simulink model "OpenFAST_ROSCO_LDP_FFP_MMPC"  (R2025b)
settings: Solver=ode4  StartTime=0.0  StopTime=TMax  FixedStep=DT  RelTol=1e-3
values from neighbouring files (symbols this model uses):
  P = P_horizon    (= 12)    [GetMPC.m]    (also in RunExample_Simulink.m = ReadWrite_FAST(fast))
undefined symbols (not defined in the file or in its folder): F, GetFASTPar, LDP, OutList, R, simu, strmatch
libraries: simulink x1
settings Model: LastModifiedBy=Aravind
settings OptimizationCC: BlockReduction=off  BooleanDataType=off
settings DebuggingCC: SaveWithParameterizedLinksMsg=none  UnderspecifiedInitializationDetection=Classic  MergeDetectMultiDrivingBlocksExec=none  SignalResolutionControl=TryResolveAllWithWarning  UnconnectedInputMsg=warning  UnconnectedOutputMsg=warning  UnconnectedLineMsg=warning
settings HardwareCC: TargetUnknown=on
settings ModelReferenceCC: EnableRefExpFcnMdlSchedulingChecks=on  PropagateSignalLabelsOutOfModel=off
settings RTWCC: GPUComputeCapability=3.5  DLArmComputeVersion=19.05

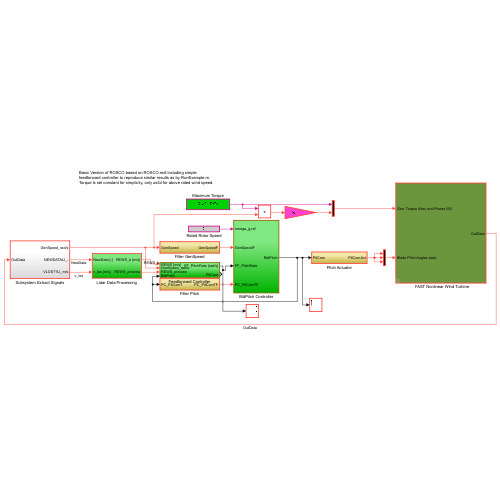
[thumbnail: Simulink's stored preview of the top-level diagram]
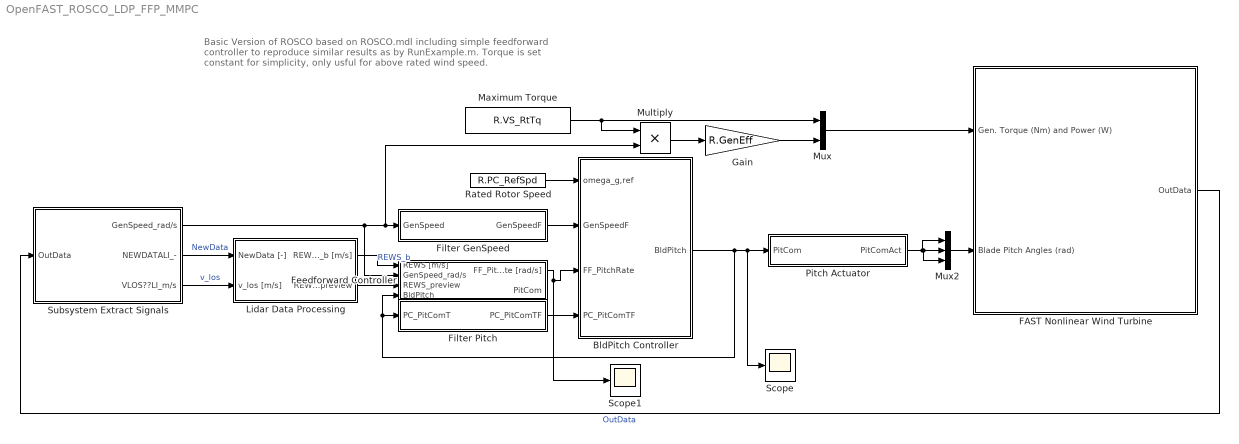
== system OpenFAST_ROSCO_LDP_FFP_MMPC ==
  note: Basic Version of ROSCO based on ROSCO.mdl including simple feedforward controller to reproduce similar results as by RunExample.m.
      | Torque is set constant for simplicity, only usful for above rated wind speed.
  "  FAST Nonlinear Wind Turbine" : Subsystem  mask(FAST Nonlinear Wind Turbine){}
      mask help: This block contains the FAST S-Function.
      mask init:
      | clear FAST_SFunc
  BldPitch Controller : Subsystem
  Feedforward Controller : Subsystem
  Filter GenSpeed : Subsystem
  Filter Pitch : Subsystem
  Gain : Gain  Gain=R.GenEff
  Lidar Data Processing : Subsystem
  Maximum Torque : Constant  Value=R.VS_RtTq
  Multiply : Product
  Mux : Mux  Inputs=2
  Mux2 : Mux  Inputs=3
  Pitch Actuator : Subsystem
  Rated Rotor Speed : Constant  Value=R.PC_RefSpd
  Scope : Scope
      settings: ActiveDisplayYMinimum=0.10219557470092069  ActiveDisplayYMaximum=0.28374092116775795  DataLoggingVariableName=ScopeData7
  Scope1 : Scope
      settings: ActiveDisplayYMinimum=-4.5750000000000979  ActiveDisplayYMaximum=4.5750000000000979  DataLoggingVariableName=ScopeData8
  Subsystem Extract Signals : Subsystem
  wires:
  Mux2/1 -> "  FAST Nonlinear Wind Turbine"/2(Blade Pitch Angles (rad))
  Rated Rotor Speed/1 -> BldPitch Controller/1(omega_g,ref)
  Subsystem Extract Signals/1(GenSpeed_rad/s) -> Feedforward Controller/2(GenSpeed_rad/s), Multiply/2, Filter GenSpeed/1(GenSpeed)
  Maximum Torque/1 -> Mux/1, Multiply/1
  Filter GenSpeed/1(GenSpeedF) -> BldPitch Controller/2(GenSpeedF)
  Gain/1 -> Mux/2
  Mux/1 -> "  FAST Nonlinear Wind Turbine"/1(Gen. Torque (Nm) and Power (W))
  Multiply/1 -> Gain/1
  "  FAST Nonlinear Wind Turbine"/1(OutData) -> Subsystem Extract Signals/1(OutData)  "OutData"
  Filter Pitch/1(PC_PitComTF) -> BldPitch Controller/4(PC_PitComTF)
  Pitch Actuator/1(PitComAct) -> Mux2/1, Mux2/3, Mux2/2
  Feedforward Controller/1(FF_PitchRate [rad/s]) -> Scope1/1, BldPitch Controller/3(FF_PitchRate)
  Subsystem Extract Signals/3(VLOS??LI_m/s) -> Lidar Data Processing/2(v_los [m/s])  "v_los"
  Lidar Data Processing/1(REWS_b [m/s]) -> Feedforward Controller/1(REWS [m/s])  "REWS_b"
  Subsystem Extract Signals/2(NEWDATALI_-) -> Lidar Data Processing/1(NewData [-])  "NewData"
  BldPitch Controller/1(BldPitch) -> Pitch Actuator/1(PitCom), Scope/1, Feedforward Controller/4(BldPitch), Filter Pitch/1(PC_PitComT)
  Lidar Data Processing/2(REWS_preview) -> Feedforward Controller/3(REWS_preview)

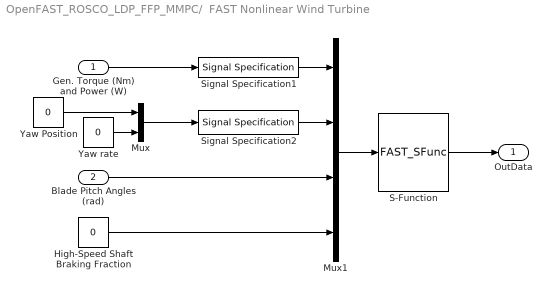
== system OpenFAST_ROSCO_LDP_FFP_MMPC/  FAST Nonlinear Wind Turbine ==
  Gen. Torque (Nm) and Power (W) : Inport
  Blade Pitch Angles (rad) : Inport  Port=2
  High-Speed Shaft Braking Fraction : Constant  Value=0
  Mux : Mux  Inputs=2
  Mux1 : Mux
  S-Function : S-Function  FunctionName=FAST_SFunc  Parameters=FAST_InputFileName, TMax, 0  SFunctionDeploymentMode=off  EnableBusSupport=off
  Signal Specification1 : SignalSpecification  OutDataTypeStr=double  Dimensions=2
  Signal Specification2 : SignalSpecification  OutDataTypeStr=double  Dimensions=2
  Yaw Position : Constant  Value=0
  Yaw rate : Constant  Value=0
  OutData : Outport
  wires:
  Gen. Torque (Nm) and Power (W)/1 -> Signal Specification1/1
  S-Function/1 -> OutData/1
  Mux1/1 -> S-Function/1
  Blade Pitch Angles (rad)/1 -> Mux1/3
  Signal Specification1/1 -> Mux1/1
  Signal Specification2/1 -> Mux1/2
  High-Speed Shaft Braking Fraction/1 -> Mux1/4
  Yaw rate/1 -> Mux/2
  Mux/1 -> Signal Specification2/1
  Yaw Position/1 -> Mux/1

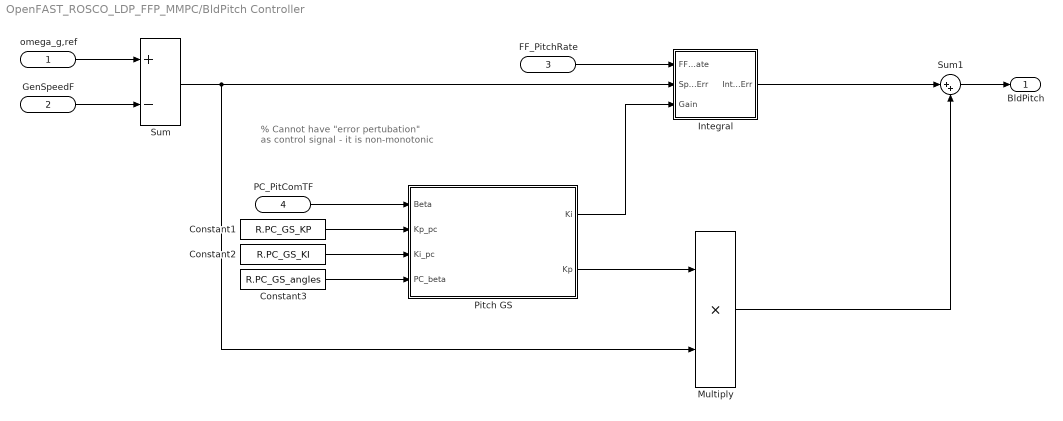
== system OpenFAST_ROSCO_LDP_FFP_MMPC/BldPitch Controller ==
  note: % Cannot have "error pertubation" as control signal
      | - it is non-monotonic
  omega_g,ref : Inport
  GenSpeedF : Inport  Port=2
  FF_PitchRate : Inport  Port=3
  PC_PitComTF : Inport  Port=4
  Constant1 : Constant  Value=R.PC_GS_KP
  Constant2 : Constant  Value=R.PC_GS_KI
  Constant3 : Constant  Value=R.PC_GS_angles
  Integral : Subsystem
  Multiply : Product
  Pitch GS : MATLAB Function  TreatAsAtomicUnit=on
  Sum : Sum  Inputs=+-
  Sum1 : Sum  Inputs=|++
  BldPitch : Outport  VectorParamsAs1DForOutWhenUnconnected=off
  wires:
  Pitch GS/1(Ki) -> Integral/3(Gain)
  omega_g,ref/1 -> Sum/1
  GenSpeedF/1 -> Sum/2
  Constant1/1 -> Pitch GS/2(Kp_pc)
  Constant2/1 -> Pitch GS/3(Ki_pc)
  Constant3/1 -> Pitch GS/4(PC_beta)
  Sum/1 -> Multiply/2, Integral/2(SpeedErr)
  Multiply/1 -> Sum1/2
  Integral/1(IntSpdErr) -> Sum1/1
  Sum1/1 -> BldPitch/1
  PC_PitComTF/1 -> Pitch GS/1(Beta)
  FF_PitchRate/1 -> Integral/1(FF_PitchRate)
  Pitch GS/2(Kp) -> Multiply/1

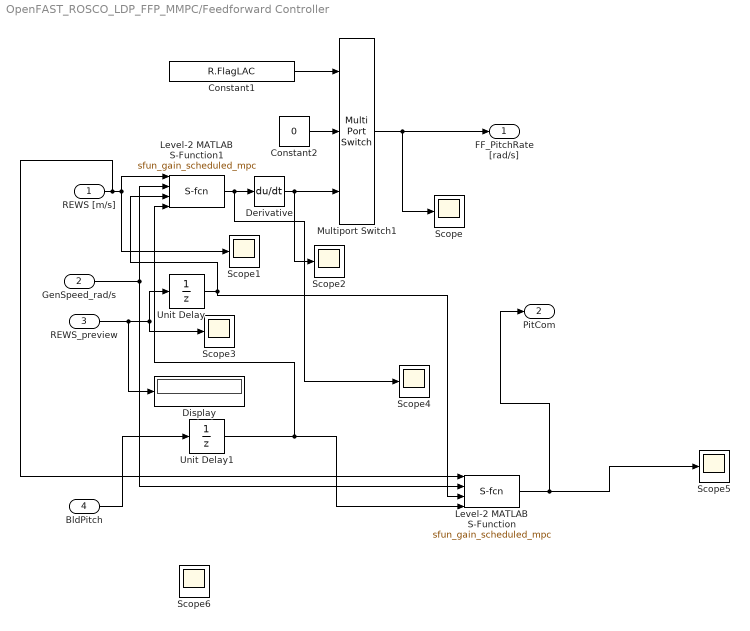
== system OpenFAST_ROSCO_LDP_FFP_MMPC/Feedforward Controller ==
  REWS [m/s] : Inport
  GenSpeed_rad/s : Inport  Port=2
  REWS_preview : Inport  Port=3
  BldPitch : Inport  Port=4
  Constant1 : Constant  Value=R.FlagLAC
  Constant2 : Constant  Value=0
  Derivative : Derivative
  Display : Display
  Level-2 MATLAB S-Function : M-S-Function  FunctionName=sfun_gain_scheduled_mpc
  Level-2 MATLAB S-Function1 : M-S-Function  FunctionName=sfun_gain_scheduled_mpc
  Multiport Switch1 : MultiPortSwitch  DataPortOrder=Specify indices  Inputs=2  DataPortIndices={0,1}  SaturateOnIntegerOverflow=off  InputSameDT=off
  Scope{,1..6} (7 alike) : Scope
      Scope settings: ActiveDisplayYMinimum=-1  ActiveDisplayYMaximum=1
      Scope1 settings: ActiveDisplayYMinimum=11.456487567346162  ActiveDisplayYMaximum=18.381466486088822  DataLoggingVariableName=ScopeData3
      Scope2 settings: ActiveDisplayYMinimum=-4.318116348637111  ActiveDisplayYMaximum=24.176537439845262  DataLoggingVariableName=ScopeData4
      Scope3 settings: ActiveDisplayYMinimum=6.7699074233965248  ActiveDisplayYMaximum=17.93615464129396  DataLoggingVariableName=ScopeData5
      Scope4 settings: ActiveDisplayYMinimum=0.080794857234064738  ActiveDisplayYMaximum=0.28427885429489819  DataLoggingVariableName=ScopeData6
      Scope5 settings: DataLoggingVariableName=ScopeData9
      Scope6 settings: DataLoggingVariableName=ScopeData10
  Unit Delay : UnitDelay  SampleTime=-1  HasFrameUpgradeWarning=on
  Unit Delay1 : UnitDelay  InitialCondition=0.1276  SampleTime=0.01  HasFrameUpgradeWarning=on
  FF_PitchRate [rad/s] : Outport  VectorParamsAs1DForOutWhenUnconnected=off
  PitCom : Outport  Port=2
  wires:
  Multiport Switch1/1 -> Scope/1, FF_PitchRate [rad/s]/1
  Constant1/1 -> Multiport Switch1/1
  Constant2/1 -> Multiport Switch1/2
  REWS [m/s]/1 -> Level-2 MATLAB S-Function/1, Level-2 MATLAB S-Function1/1, Scope1/1
  Derivative/1 -> Scope2/1, Multiport Switch1/3
  Level-2 MATLAB S-Function1/1 -> Scope4/1, Derivative/1
  GenSpeed_rad/s/1 -> Level-2 MATLAB S-Function/2, Level-2 MATLAB S-Function1/2
  REWS_preview/1 -> Scope3/1, Unit Delay/1, Display/1
  Unit Delay/1 -> Level-2 MATLAB S-Function1/3, Level-2 MATLAB S-Function/3
  BldPitch/1 -> Unit Delay1/1
  Level-2 MATLAB S-Function/1 -> PitCom/1, Scope5/1
  Unit Delay1/1 -> Level-2 MATLAB S-Function1/4, Level-2 MATLAB S-Function/4

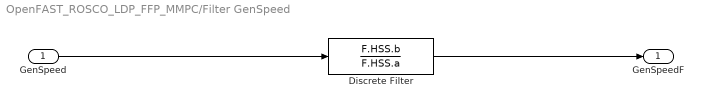
== system OpenFAST_ROSCO_LDP_FFP_MMPC/Filter GenSpeed ==
  GenSpeed : Inport
  Discrete Filter : DiscreteFilter  Numerator=F.HSS.b  Denominator=F.HSS.a  InitialStates=R.PC_RefSpd/(sum(F.HSS.a(2:end))+1)
  GenSpeedF : Outport  VectorParamsAs1DForOutWhenUnconnected=off
  wires:
  Discrete Filter/1 -> GenSpeedF/1
  GenSpeed/1 -> Discrete Filter/1

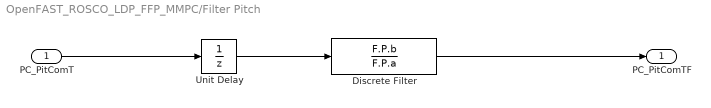
== system OpenFAST_ROSCO_LDP_FFP_MMPC/Filter Pitch ==
  PC_PitComT : Inport
  Discrete Filter : DiscreteFilter  Numerator=F.P.b  Denominator=F.P.a
  Unit Delay : UnitDelay  SampleTime=-1  HasFrameUpgradeWarning=on
  PC_PitComTF : Outport  VectorParamsAs1DForOutWhenUnconnected=off
  wires:
  PC_PitComT/1 -> Unit Delay/1
  Discrete Filter/1 -> PC_PitComTF/1
  Unit Delay/1 -> Discrete Filter/1

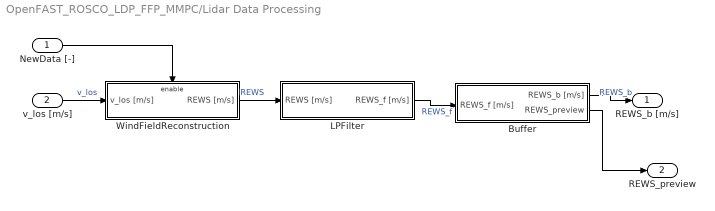
== system OpenFAST_ROSCO_LDP_FFP_MMPC/Lidar Data Processing ==
  NewData [-] : Inport
  v_los [m/s] : Inport  Port=2
  Buffer : Subsystem
  LPFilter : Subsystem
  WindFieldReconstruction : Subsystem
  REWS_b [m/s] : Outport  VectorParamsAs1DForOutWhenUnconnected=off
  REWS_preview : Outport  Port=2
  wires:
  v_los [m/s]/1 -> WindFieldReconstruction/1(v_los [m/s])  "v_los"
  NewData [-]/1 -> WindFieldReconstruction/Enable
  Buffer/1(REWS_b [m/s]) -> REWS_b [m/s]/1  "REWS_b"
  WindFieldReconstruction/1(REWS [m/s]) -> LPFilter/1(REWS [m/s])  "REWS"
  LPFilter/1(REWS_f [m/s]) -> Buffer/1(REWS_f [m/s])  "REWS_f"
  Buffer/2(REWS_preview) -> REWS_preview/1

== system OpenFAST_ROSCO_LDP_FFP_MMPC/Pitch Actuator ==
  PitCom : Inport
  Discrete Filter : DiscreteFilter  Numerator=F.F_PitchAct.b  Denominator=F.F_PitchAct.a  InitialStates=GetFASTPar(P.EDP,'BlPitch(1)')/180*pi/(sum(F.F_PitchAct.a(2:end))+1)
  PitComAct : Outport  VectorParamsAs1DForOutWhenUnconnected=off
  wires:
  PitCom/1 -> Discrete Filter/1
  Discrete Filter/1 -> PitComAct/1

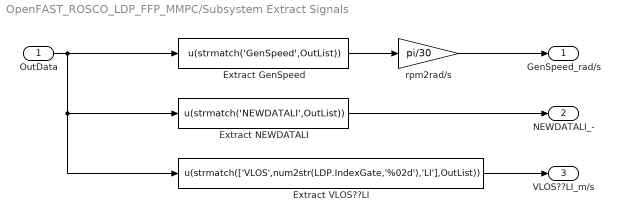
== system OpenFAST_ROSCO_LDP_FFP_MMPC/Subsystem Extract Signals ==
  OutData : Inport
  Extract GenSpeed : Fcn  Expr=u(strmatch('GenSpeed',OutList))
  Extract NEWDATALI : Fcn  Expr=u(strmatch('NEWDATALI',OutList))
  Extract VLOS??LI : Fcn  Expr=u(strmatch(['VLOS',num2str(LDP.IndexGate,'%02d'),'LI'],OutList))
  rpm2rad/s : Gain  Gain=pi/30
  GenSpeed_rad/s : Outport  VectorParamsAs1DForOutWhenUnconnected=off
  NEWDATALI_- : Outport  Port=2  VectorParamsAs1DForOutWhenUnconnected=off
  VLOS??LI_m/s : Outport  Port=3  VectorParamsAs1DForOutWhenUnconnected=off
  wires:
  rpm2rad/s/1 -> GenSpeed_rad/s/1
  Extract GenSpeed/1 -> rpm2rad/s/1
  OutData/1 -> Extract GenSpeed/1, Extract NEWDATALI/1, Extract VLOS??LI/1
  Extract VLOS??LI/1 -> VLOS??LI_m/s/1
  Extract NEWDATALI/1 -> NEWDATALI_-/1

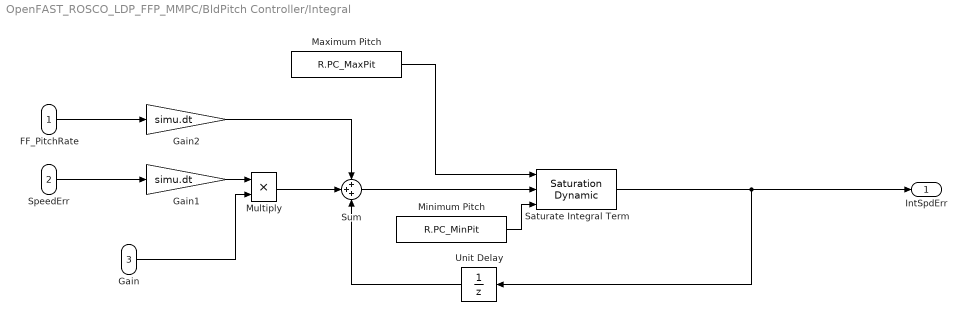
== system OpenFAST_ROSCO_LDP_FFP_MMPC/BldPitch Controller/Integral ==
  FF_PitchRate : Inport
  SpeedErr : Inport  Port=2
  Gain : Inport  Port=3
  Gain1 : Gain  Gain=simu.dt
  Gain2 : Gain  Gain=simu.dt
  Maximum Pitch : Constant  Value=R.PC_MaxPit
  Minimum Pitch : Constant  Value=R.PC_MinPit
  Multiply : Product
  Saturate Integral Term : simulink/Discontinuities/Saturation Dynamic  OutMin=[]  OutMax=[]  OutDataTypeStr=Inherit: Same as second input  OutDataType=fixdt(1, 16)  OutScaling=2^-10  RndMeth=Nearest  DoSatur=off
  Sum : Sum  Inputs=+++
  Unit Delay : UnitDelay  InitialCondition=GetFASTPar(P.EDP,'BlPitch(1)')/180*pi  SampleTime=-1  HasFrameUpgradeWarning=on
  IntSpdErr : Outport  VectorParamsAs1DForOutWhenUnconnected=off
  wires:
  Maximum Pitch/1 -> Saturate Integral Term/1
  Sum/1 -> Saturate Integral Term/2
  SpeedErr/1 -> Gain1/1
  Gain/1 -> Multiply/2
  Saturate Integral Term/1 -> IntSpdErr/1, Unit Delay/1
  Gain1/1 -> Multiply/1
  Minimum Pitch/1 -> Saturate Integral Term/3
  Unit Delay/1 -> Sum/3
  Multiply/1 -> Sum/2
  Gain2/1 -> Sum/1
  FF_PitchRate/1 -> Gain2/1

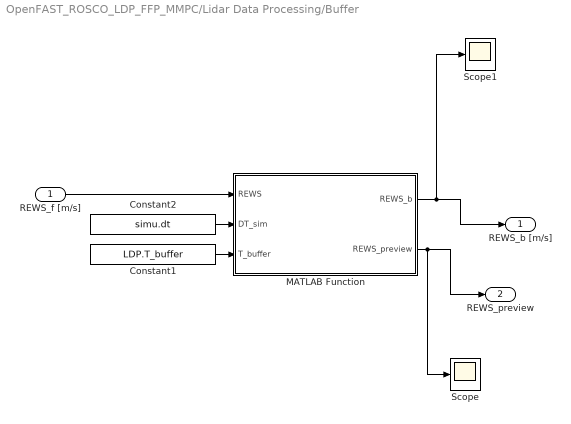
== system OpenFAST_ROSCO_LDP_FFP_MMPC/Lidar Data Processing/Buffer ==
  REWS_f [m/s] : Inport
  Constant1 : Constant  Value=LDP.T_buffer
  Constant2 : Constant  Value=simu.dt
  MATLAB Function : MATLAB Function  TreatAsAtomicUnit=on
  Scope : Scope
      settings: ActiveDisplayYMinimum=-1  ActiveDisplayYMaximum=1
  Scope1 : Scope
      settings: ActiveDisplayYMinimum=11.514550147546224  ActiveDisplayYMaximum=18.388313377142136  DataLoggingVariableName=ScopeData2
  REWS_b [m/s] : Outport  VectorParamsAs1DForOutWhenUnconnected=off
  REWS_preview : Outport  Port=2
  wires:
  Constant1/1 -> MATLAB Function/3(T_buffer)
  Constant2/1 -> MATLAB Function/2(DT_sim)
  REWS_f [m/s]/1 -> MATLAB Function/1(REWS)
  MATLAB Function/2(REWS_preview) -> Scope/1, REWS_preview/1
  MATLAB Function/1(REWS_b) -> Scope1/1, REWS_b [m/s]/1

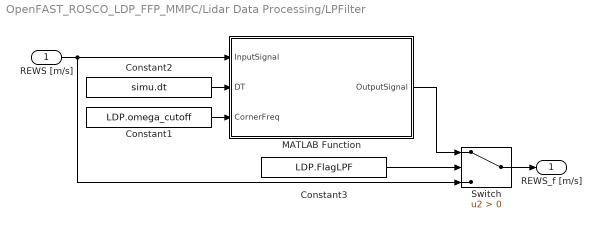
== system OpenFAST_ROSCO_LDP_FFP_MMPC/Lidar Data Processing/LPFilter ==
  REWS [m/s] : Inport
  Constant1 : Constant  Value=LDP.omega_cutoff
  Constant2 : Constant  Value=simu.dt
  Constant3 : Constant  Value=LDP.FlagLPF
  MATLAB Function : MATLAB Function  TreatAsAtomicUnit=on
  Switch : Switch  Criteria=u2 > Threshold  SaturateOnIntegerOverflow=off  InputSameDT=off
  REWS_f [m/s] : Outport  VectorParamsAs1DForOutWhenUnconnected=off
  wires:
  REWS [m/s]/1 -> MATLAB Function/1(InputSignal), Switch/3
  Constant2/1 -> MATLAB Function/2(DT)
  Constant1/1 -> MATLAB Function/3(CornerFreq)
  Switch/1 -> REWS_f [m/s]/1
  Constant3/1 -> Switch/2
  MATLAB Function/1(OutputSignal) -> Switch/1

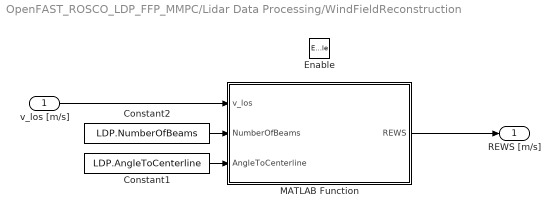
== system OpenFAST_ROSCO_LDP_FFP_MMPC/Lidar Data Processing/WindFieldReconstruction ==
  v_los [m/s] : Inport
  Enable : EnablePort
  Constant1 : Constant  Value=LDP.AngleToCenterline
  Constant2 : Constant  Value=LDP.NumberOfBeams
  MATLAB Function : MATLAB Function  TreatAsAtomicUnit=on
  REWS [m/s] : Outport  VectorParamsAs1DForOutWhenUnconnected=off
  wires:
  MATLAB Function/1(REWS) -> REWS [m/s]/1
  v_los [m/s]/1 -> MATLAB Function/1(v_los)
  Constant2/1 -> MATLAB Function/2(NumberOfBeams)
  Constant1/1 -> MATLAB Function/3(AngleToCenterline)

== matlab function OpenFAST_ROSCO_LDP_FFP_MMPC/Lidar Data Processing/Buffer/MATLAB Function ==
  data: REWS input; REWS_b output size=1; DT_sim input; T_buffer input; REWS_preview output size=551
function [REWS_b, REWS_preview] = Buffer(REWS, DT_sim, T_buffer)
%#codegen
Np               = 550;
nPreviewElements = 551;
nBuffer          = 2000;
FREEZE_SAMPLES   = round(5.5 / DT_sim);   % 550 at 0.01 s

persistent REWS_f_Buffer;
if isempty(REWS_f_Buffer)
    REWS_f_Buffer = ones(nBuffer, 1, 'double') * 12.5;
end

REWS_double   = double(REWS);
REWS_f_Buffer = [REWS_double; REWS_f_Buffer(1:nBuffer-1)];

Idx_now = min(max(floor(T_buffer/DT_sim) + 1, 1), nBuffer);
REWS_b  = REWS_f_Buffer(Idx_now);

REWS_preview = zeros(nPreviewElements, 1, 'double');
if Idx_now >= nPreviewElements
    REWS_preview(:) = flip(REWS_f_Buffer(Idx_now - Np : Idx_now));
else
    available = Idx_now;
    REWS_preview(1:available)       = flip(REWS_f_Buffer(1:Idx_now));
    REWS_preview(available+1 : end) = REWS_f_Buffer(1);
end

% Hardcode both outputs to 12.5 for the first 5.5 seconds
% Idx_now counts samples pushed into buffer — at 0.01 s, 5.5 s = 550 samples
if Idx_now <= FREEZE_SAMPLES
    REWS_b           = 12.5;
    REWS_preview(:)  = 12.5;
end

end

== matlab function OpenFAST_ROSCO_LDP_FFP_MMPC/Lidar Data Processing/WindFieldReconstruction/MATLAB Function ==
  data: v_los input; REWS output; NumberOfBeams input; AngleToCenterline input
function REWS = WindFieldReconstruction(v_los,NumberOfBeams,AngleToCenterline)
% matlab version of the subroutine WindFieldReconstruction in LDP_v1_Subs.f90

% init u_est_Buffer
persistent u_est_Buffer;
if isempty(u_est_Buffer)      
    u_est_Buffer = NaN(NumberOfBeams,1);   
end 

% Estimate u component assuming perfect alignment
u_est 		    = v_los/cosd(AngleToCenterline);

% Update Buffer for estimated u component
u_est_Buffer    = [u_est;u_est_Buffer(1:NumberOfBeams-1)];

% Calculate REWS from mean over all estimated u components
REWS  	        = mean(u_est_Buffer,'omitnan');

end

== matlab function OpenFAST_ROSCO_LDP_FFP_MMPC/Lidar Data Processing/LPFilter/MATLAB Function ==
  data: InputSignal input; OutputSignal output; DT input; CornerFreq input
function OutputSignal = LPFilter(InputSignal,DT,CornerFreq)
% matlab version of the function LPFilter in FFP_v1_Subs.f90

% Initialization
persistent OutputSignalLast InputSignalLast;
if isempty(OutputSignalLast)      
    OutputSignalLast    = InputSignal;  
    InputSignalLast     = InputSignal;
end 

% Define coefficients 
a1          = 2 + CornerFreq*DT;
a0          = CornerFreq*DT - 2;
b1          = CornerFreq*DT;
b0          = CornerFreq*DT;

% Filter
OutputSignal = 1.0/a1 * (-a0*OutputSignalLast + b1*InputSignal + b0*InputSignalLast);

% Save signals for next time step
InputSignalLast     = InputSignal;
OutputSignalLast    = OutputSignal;
end

== matlab function OpenFAST_ROSCO_LDP_FFP_MMPC/BldPitch Controller/Pitch GS ==
  data: Ki output size=1; Beta input; Kp_pc input; Kp output size=1; Ki_pc input; PC_beta input
 function [Ki, Kp] = GainSchedule(Beta, Kp_pc, Ki_pc,  PC_beta)

% This function calculates the current gains for a Collective Blade Pitch 
% controller
%
% Inputs: v - Current wind speed estimate, m/s.
%         ContParam - Structure of control parameters, output from
%                     ControlParameters.m
%
% Outputs: Kp - Proportional Gain
%          Ki - Integral Gain
%
% Nikhar Abbas - May 2019


%% Linear Gain Schedule
% pKp_pc = ContParam.GS.pKp_pc;
% pKi_pc = ContParam.GS.pKi_pc;
% 
% %%
% Kp = pKp_pc(1)*Beta + pKp_pc(2);
% Ki = pKi_pc(1)*Beta + pKi_pc(2);
% % Kp = pKp_pc(1)*v + pKp_pc(2)
% % Ki = pKi_pc(1)*v + pKi_pc(2);
% 
% Kpmax = pKp_pc(1)*15*pi/180 + pKp_pc(2);
% Kimax = pKi_pc(1)*15*pi/180 + pKi_pc(2);
% 
% Kp = min(Kp, Kpmax);
% Ki = min(Ki,Kimax);

%% nonlinear Gain Schedule
% Kp_pc   = R.PC_GS_KP;
% Ki_pc   = R.PC_GS_KI;
% PC_beta = R.PC_GS_angles;

beta    = max(min(Beta,PC_beta(end)), PC_beta(1));

% gains
Kp      = interp1(PC_beta,Kp_pc, beta);
Ki      = interp1(PC_beta,Ki_pc, beta);



end
